simulink model "Drone_model"  (R2021a)
settings: Solver=VariableStepAuto  StartTime=0.0  StopTime=10.0  RelTol=1e-3
undefined symbols (not defined in the file): b, d
settings Model: Creator=Dell  LastModifiedBy=Dell

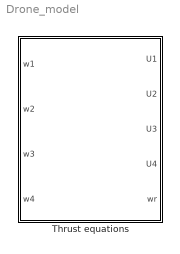
== system Drone_model ==
  Thrust equations : Subsystem

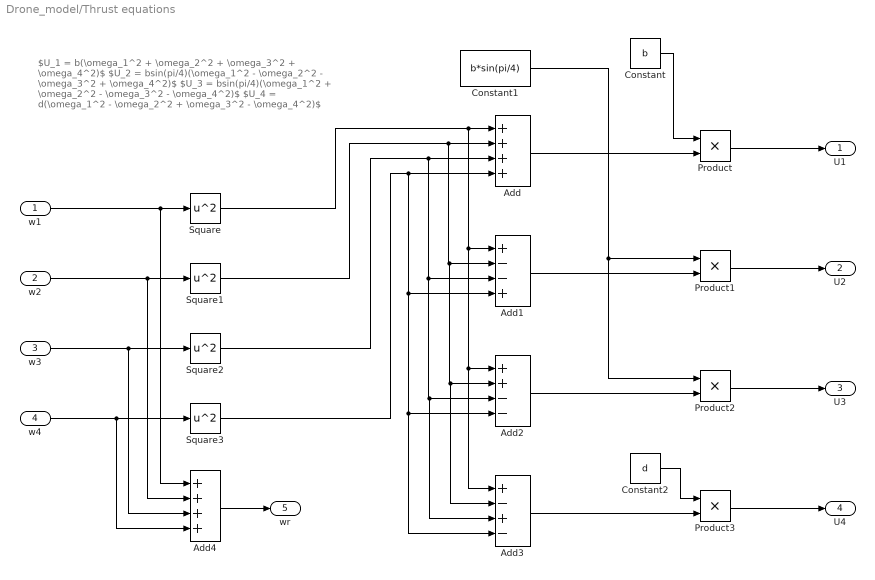
== system Drone_model/Thrust equations ==
  note: $U_1 = b(\omega_1^2 + \omega_2^2 + \omega_3^2 + \omega_4^2)$
      | $U_2 = bsin(pi/4)(\omega_1^2 - \omega_2^2 - \omega_3^2 + \omega_4^2)$
      | $U_3 = bsin(pi/4)(\omega_1^2 + \omega_2^2 - \omega_3^2 - \omega_4^2)$
      | $U_4 = d(\omega_1^2 - \omega_2^2 + \omega_3^2 - \omega_4^2)$
  w1 : Inport
  w2 : Inport  Port=2
  w3 : Inport  Port=3
  w4 : Inport  Port=4
  Add : Sum  Inputs=++++
  Add1 : Sum  Inputs=+--+
  Add2 : Sum  Inputs=++--
  Add3 : Sum  Inputs=+-+-
  Add4 : Sum  Inputs=++++
  Constant : Constant  Value=b
  Constant1 : Constant  Value=b*sin(pi/4)
  Constant2 : Constant  Value=d
  Product{,1..3} (4 alike) : Product
  Square{,1..3} (4 alike) : Math  Operator=square  SaturateOnIntegerOverflow=on
  U1 : Outport
  U2 : Outport  Port=2
  U3 : Outport  Port=3
  U4 : Outport  Port=4
  wr : Outport  Port=5
  wires:
  w1/1 -> Add4/1, Square/1
  w2/1 -> Add4/2, Square1/1
  w3/1 -> Add4/3, Square2/1
  w4/1 -> Add4/4, Square3/1
  Square/1 -> Add3/1, Add2/1, Add1/1, Add/1
  Square1/1 -> Add3/2, Add2/2, Add1/2, Add/2
  Square2/1 -> Add3/3, Add2/3, Add1/3, Add/3
  Square3/1 -> Add2/4, Add3/4, Add1/4, Add/4
  Product/1 -> U1/1
  Product1/1 -> U2/1
  Product2/1 -> U3/1
  Product3/1 -> U4/1
  Add/1 -> Product/2
  Add1/1 -> Product1/2
  Add2/1 -> Product2/2
  Add3/1 -> Product3/2
  Constant/1 -> Product/1
  Constant1/1 -> Product2/1, Product1/1
  Constant2/1 -> Product3/1
  Add4/1 -> wr/1
